simulink model "sp2_2"  (R2020b)
settings: Solver=VariableStepAuto  StartTime=0.0  StopTime=5  MaxStep=0.01  RelTol=1e-3
settings Model: Creator=seojoon  LastModifiedBy=seojoon
settings DataIOCC: ReturnWorkspaceOutputs=off

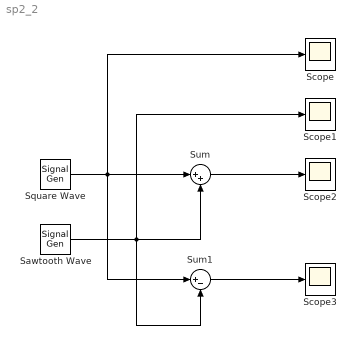
== system sp2_2 ==
  Sawtooth Wave : SignalGenerator  WaveForm=sawtooth  Amplitude=0.5  Frequency=0.5
  Scope{,1..3} (4 alike) : Scope
  Square Wave : SignalGenerator  WaveForm=square
  Sum : Sum  Inputs=|++
  Sum1 : Sum  Inputs=|+-
  wires:
  Sum1/1 -> Scope3/1
  Sum/1 -> Scope2/1
  Square Wave/1 -> Scope/1, Sum1/1, Sum/1
  Sawtooth Wave/1 -> Sum/2, Sum1/2, Scope1/1
